simulink model "Exercise31"  (R2016a)
settings: Solver=VariableStepAuto  StartTime=0.0  StopTime=10.0  RelTol=1e-3
values from neighbouring files (symbols this model uses):
  Fh = 10.39*1e6    (= 10390000)    [Exercise3.m]
  Fl = 10.21*1e6    (= 10210000)    [Exercise3.m]
  Ts = 1/Fs    (= 2.77777777778e-06)    [Exercise3.m]
settings Model: Creator=sergi  LastModifiedBy=sergi

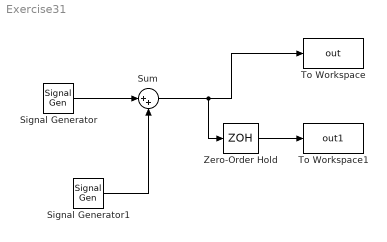
== system Exercise31 ==
  Signal Generator : SignalGenerator  Frequency=Fl
  Signal Generator1 : SignalGenerator  Frequency=Fh
  Sum : Sum  Inputs=|++
  To Workspace : ToWorkspace  VariableName=out  SampleTime=Ts/10
      settings: Save2DSignal=2-D array (concatenate along first dimension)
  To Workspace1 : ToWorkspace  VariableName=out1  SampleTime=Ts/10
      settings: Save2DSignal=2-D array (concatenate along first dimension)
  Zero-Order Hold : ZeroOrderHold  SampleTime=Ts
  wires:
  Zero-Order Hold/1 -> To Workspace1/1
  Signal Generator/1 -> Sum/1
  Signal Generator1/1 -> Sum/2
  Sum/1 -> Zero-Order Hold/1, To Workspace/1
